simulink model "mhk_vanderpol_8am"  (Simulink 7.5)
settings: Solver=ode45  StartTime=0.0  StopTime=30  RelTol=1e-3
settings Model: Creator=mhkeme  LastModifiedBy=mhkeme

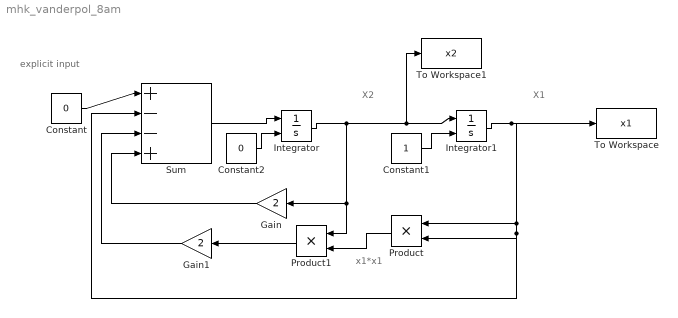
== system mhk_vanderpol_8am ==
  note: X2
  note: X1
  note: explicit input
  note: x1*x1
  Constant : Constant  Value=0  OutDataType=fixdt(1, 16)  OutScaling=2^0
  Constant1 : Constant  OutDataType=fixdt(1, 16)  OutScaling=2^0
  Constant2 : Constant  Value=0  OutDataType=fixdt(1, 16)  OutScaling=2^0
  Gain : Gain  Gain=2  ParameterDataType=fixdt(1, 16)  ParameterScaling=2^0  OutDataType=fixdt(1, 16)  OutScaling=2^0
  Gain1 : Gain  Gain=2  ParameterDataType=fixdt(1, 16)  ParameterScaling=2^0  OutDataType=fixdt(1, 16)  OutScaling=2^0
  Integrator : Integrator  InitialConditionSource=external
  Integrator1 : Integrator  InitialConditionSource=external
  Product : Product  OutDataType=fixdt(1, 16)  OutScaling=2^0  RndMeth=Zero
  Product1 : Product  OutDataType=fixdt(1, 16)  OutScaling=2^0  RndMeth=Zero
  Sum : Sum  Inputs=|+--+  OutDataType=fixdt(1, 16)  OutScaling=2^0
  To Workspace : ToWorkspace  VariableName=x1  SampleTime=-1  SaveFormat=Array
  To Workspace1 : ToWorkspace  VariableName=x2  SampleTime=-1  SaveFormat=Array
  wires:
  Integrator/1 -> Gain/1, Product1/1, Integrator1/1, To Workspace1/1
  Sum/1 -> Integrator/1
  Constant/1 -> Sum/1
  Gain/1 -> Sum/4
  Integrator1/1 -> Product/1, Product/2, Sum/2, To Workspace/1
  Product/1 -> Product1/2
  Product1/1 -> Gain1/1
  Gain1/1 -> Sum/3
  Constant1/1 -> Integrator1/2
  Constant2/1 -> Integrator/2
